simulink model "untitled"  (R2023b)
settings: Solver=VariableStepAuto  StartTime=0.0  StopTime=30  RelTol=1e-3
InitFcn:
  | clc;
  | 
  | I_xx = 228.211;
  | I_yy = 228.211;
  | I_zz = 246.355;
  | 
  | 
  | 
  | m = 327.316; %mass
  | g = 9.81; %gravitational acceleration
  | p = 1.225; %density of the environment
  | 
  | 
  | %aerodynamic forces are negligible
  | C_L = 0;
  | C_D = 0;
  | 
  | 
  | %Vector from center of gravity to the
  | %center of pressure
  | r_CP = [ 0.2; 0.0; 0.0];
  | 
  | k_r = 0.0001; %Aerodynamic damping coefficient
  | 
  | c = 20; %coefficient to calculate counter-moment
  | 
  | l = 2; %Rotor moment arm length
  | 
  | T_max = 1500; %Max thrust
  | 
  | tau = 0.05;
  | 
  | v_B = [0; 0; 0];
  | 
  | w_B = [0; 0; 0];
  | 
  | x_I = [0;0; -5];
  | 
  | euler_angles = [0;0;0];
settings Model: Creator=nijatabbasov  LastModifiedBy=nijatabbasov

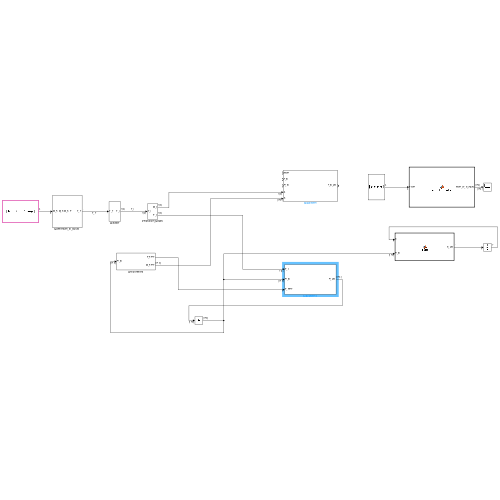
[thumbnail: Simulink's stored preview of the top-level diagram]
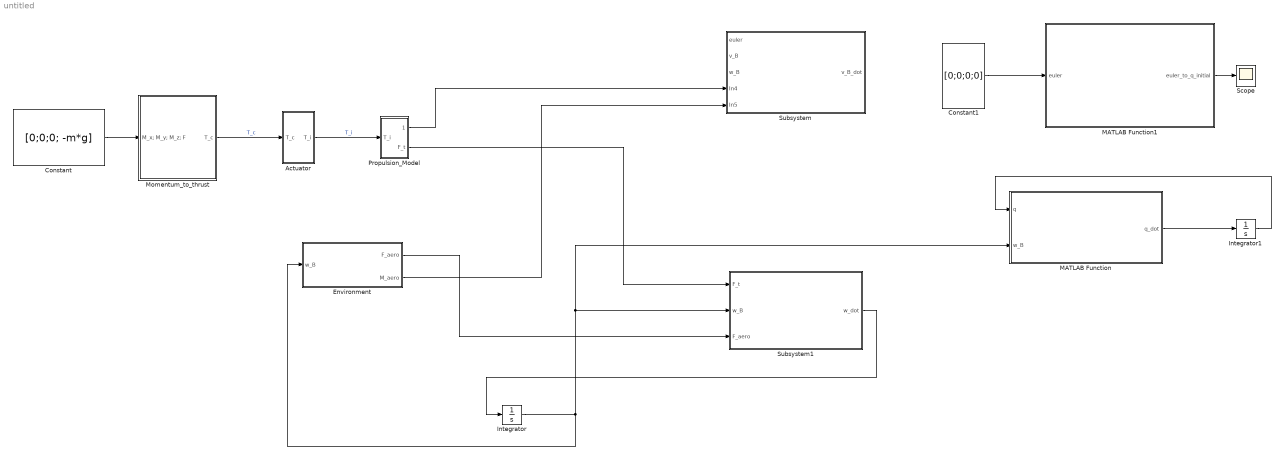
== system untitled ==
  Actuator : Subsystem
  Constant : Constant  Value=[0;0;0; -m*g]
  Constant1 : Constant  Value=[0;0;0;0]
  Environment : Subsystem
  Integrator : Integrator
  Integrator1 : Integrator
  MATLAB Function : MATLAB Function  TreatAsAtomicUnit=on
  MATLAB Function1 : MATLAB Function  TreatAsAtomicUnit=on
  "Momentum_to_thrust " : Subsystem
  Propulsion_Model : Subsystem
  Scope : Scope
  Subsystem : Subsystem
  Subsystem1 : Subsystem
  wires:
  Constant/1 -> "Momentum_to_thrust "/1(M_x; M_y; M_z; F)
  "Momentum_to_thrust "/1(T_c) -> Actuator/1(T_c)  "T_c"
  Actuator/1(T_i) -> Propulsion_Model/1(T_i)  "T_i"
  Propulsion_Model/1(M_t) -> Subsystem/4(In4)
  Environment/2(M_aero) -> Subsystem/5(In5)
  Propulsion_Model/2(F_t) -> Subsystem1/1(F_t)
  Environment/1(F_aero) -> Subsystem1/3(F_aero)
  Subsystem1/1(w_dot) -> Integrator/1
  Integrator/1 -> MATLAB Function/2(w_B), Subsystem1/2(w_B), Environment/1(w_B)
  MATLAB Function/1(q_dot) -> Integrator1/1
  Integrator1/1 -> MATLAB Function/1(q)
  Constant1/1 -> MATLAB Function1/1(euler)
  MATLAB Function1/1(euler_to_q_initial) -> Scope/1

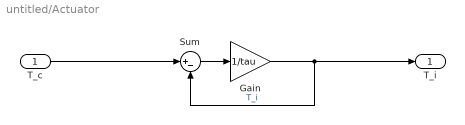
== system untitled/Actuator ==
  T_c : Inport
  Gain : Gain  Gain=1/tau
  Sum : Sum  Inputs=|+-
  T_i : Outport
  wires:
  T_c/1 -> Sum/1
  Gain/1 -> T_i/1, Sum/2  "T_i"
  Sum/1 -> Gain/1

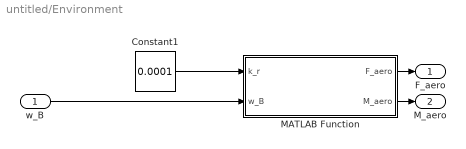
== system untitled/Environment ==
  w_B : Inport
  Constant1 : Constant  Value=0.0001
  MATLAB Function : MATLAB Function  TreatAsAtomicUnit=on
  F_aero : Outport
  M_aero : Outport  Port=2
  wires:
  w_B/1 -> MATLAB Function/2(w_B)
  MATLAB Function/2(M_aero) -> M_aero/1
  MATLAB Function/1(F_aero) -> F_aero/1
  Constant1/1 -> MATLAB Function/1(k_r)

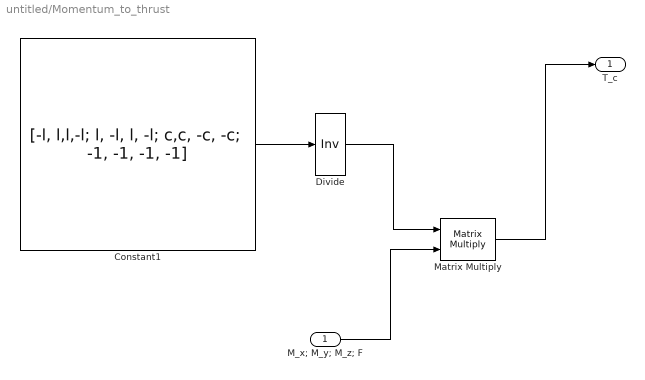
== system untitled/Momentum_to_thrust  ==
  M_x; M_y; M_z; F : Inport
  Constant1 : Constant  Value=[-l, l,l,-l; l, -l, l, -l; c,c, -c, -c; -1, -1, -1, -1]
  Divide : Product  Inputs=/  Multiplication=Matrix(*)  OutDataTypeStr=double
  Matrix Multiply : Product  Multiplication=Matrix(*)
  T_c : Outport
  wires:
  M_x; M_y; M_z; F/1 -> Matrix Multiply/2
  Matrix Multiply/1 -> T_c/1
  Divide/1 -> Matrix Multiply/1
  Constant1/1 -> Divide/1

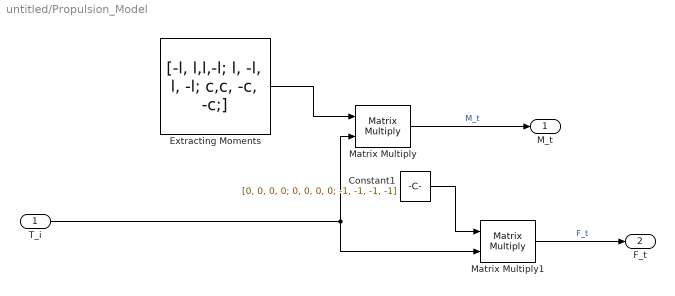
== system untitled/Propulsion_Model ==
  T_i : Inport
  Constant1 : Constant  Value=[0, 0, 0, 0; 0, 0, 0, 0; -1, -1, -1, -1]
  Extracting Moments : Constant  Value=[-l, l,l,-l; l, -l, l, -l; c,c, -c, -c;]
  Matrix Multiply : Product  Multiplication=Matrix(*)
  Matrix Multiply1 : Product  Multiplication=Matrix(*)
  M_t : Outport
  F_t : Outport  Port=2
  wires:
  T_i/1 -> Matrix Multiply1/2, Matrix Multiply/2
  Matrix Multiply/1 -> M_t/1  "M_t"
  Extracting Moments/1 -> Matrix Multiply/1
  Matrix Multiply1/1 -> F_t/1  "F_t"
  Constant1/1 -> Matrix Multiply1/1

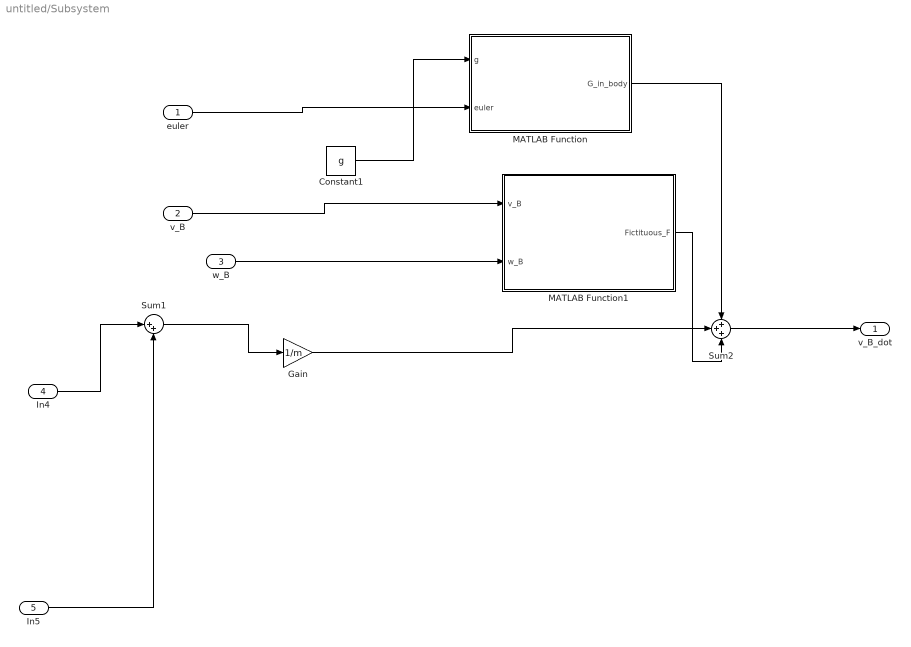
== system untitled/Subsystem ==
  euler : Inport
  v_B : Inport  Port=2
  w_B : Inport  Port=3
  In4 : Inport  Port=4
  In5 : Inport  Port=5
  Constant1 : Constant  Value=g
  Gain : Gain  Gain=1/m
  MATLAB Function : MATLAB Function  TreatAsAtomicUnit=on
  MATLAB Function1 : MATLAB Function  TreatAsAtomicUnit=on
  Sum1 : Sum  Inputs=|++
  Sum2 : Sum  Inputs=+++
  v_B_dot : Outport
  wires:
  In4/1 -> Sum1/1
  In5/1 -> Sum1/2
  w_B/1 -> MATLAB Function1/2(w_B)
  MATLAB Function/1(G_in_body) -> Sum2/1
  Constant1/1 -> MATLAB Function/1(g)
  euler/1 -> MATLAB Function/2(euler)
  MATLAB Function1/1(Fictituous_F) -> Sum2/3
  Gain/1 -> Sum2/2
  v_B/1 -> MATLAB Function1/1(v_B)
  Sum2/1 -> v_B_dot/1
  Sum1/1 -> Gain/1

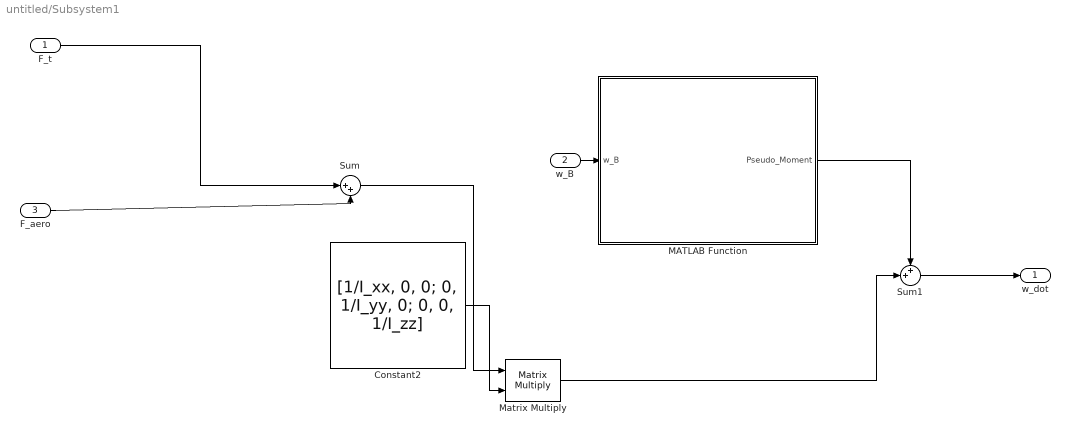
== system untitled/Subsystem1 ==
  F_t : Inport
  w_B : Inport  Port=2
  F_aero : Inport  Port=3
  Constant2 : Constant  Value=[1/I_xx, 0, 0; 0, 1/I_yy, 0; 0, 0, 1/I_zz]
  MATLAB Function : MATLAB Function  TreatAsAtomicUnit=on
  Matrix Multiply : Product  Multiplication=Matrix(*)
  Sum : Sum  Inputs=|++
  Sum1 : Sum  Inputs=++|
  w_dot : Outport
  wires:
  F_t/1 -> Sum/1
  Matrix Multiply/1 -> Sum1/2
  w_B/1 -> MATLAB Function/1(w_B)
  Constant2/1 -> Matrix Multiply/2
  Sum1/1 -> w_dot/1
  F_aero/1 -> Sum/2
  Sum/1 -> Matrix Multiply/1
  MATLAB Function/1(Pseudo_Moment) -> Sum1/1

== matlab function untitled/Subsystem/MATLAB Function ==
  data: g input; G_in_body output; euler input
function G_in_body = G_in_body(g, euler)
    % This function evaluates derivative of vehicle speed in body frame 
    % and angular velocity of the center of gravity of the vehicle
    %Acceler is (F_thrust + F_aero)/m
    phi = euler(1);
    theta = euler(2);
    

    
    frame_change = [-sin(theta); sin(phi)*cos(theta); cos(phi)* cos(theta)];


    G_in_body = frame_change * g;
   
end

== matlab function untitled/Environment/MATLAB Function ==
  data: k_r input; F_aero output; w_B input; M_aero output
function [F_aero, M_aero] = F_aero_M_aero(k_r, w_B)

    F_aero = 0;
    M_aero = - k_r * w_B;

== matlab function untitled/Subsystem/MATLAB Function1 ==
  data: v_B input; Fictituous_F output; w_B input
function Fictituous_F = Fictituous_F(v_B, w_B)
    % This function evaluates derivative of vehicle speed in body frame 
    % and angular velocity of the center of gravity of the vehicle
    
    p = w_B(1);
    q = w_B(2);
    r = w_B(3);


    w_x = [0, -r,  q;
           r,  0, -p;
          -1   p   0   ];

   

    Fictituous_F = w_x * v_B;
    
end

== matlab function untitled/Subsystem1/MATLAB Function ==
  data: w_B input; Pseudo_Moment output
function Pseudo_Moment = Pseudo_Moment(w_B)
    % This function evaluates value of w*(Iw)
   
    p = w_B(1);
    q = w_B(2);
    r = w_B(3);


    
    
   
    I_xx = 228.211; 
    I_yy = 228.211;
    I_zz = 246.355;



    Pseudo_Moment = [(I_yy-I_zz)*q*r/I_xx; (I_zz - I_xx)*p*r/I_yy; (I_xx - I_yy)*p*q/I_zz];
   
    
end

== matlab function untitled/MATLAB Function ==
  data: q input; q_dot output; w_B input
function q_dot = q_dot(q, w_B)
    q_0 = q(1);
    q_1 = q(2);
    q_2 = q(3);
    q_3 = q(4);

    p = w_B(1);
    q = w_B(2);
    r = w_B(3);

    epsilon_q = 1-(q_0^2 + q_1^2 + q_2^2 + q_3^2);

    C_k = 5;
    A = [0, -p, -q, -r;
         p,  0,  r, -q;
         q, -r,  0,  p;
         r,  q, -p,  0];

    
    q_dot = 1/2 * A *q + C_k * epsilon_q*q;


end

== matlab function untitled/MATLAB Function1 ==
  data: euler input; euler_to_q_initial output
function euler_to_q_initial = euler_to_q_initial(euler)

    phi = euler(1); 
    theta = euler(2); 
    psi = euler(3);


    phi = deg2rad(phi);
    theta = deg2rad(theta);
    psi = deg2rad(psi);

    q0 = cos(psi/2)*cos(theta/2)*cos(phi/2) + sin(psi/2)*sin(theta/2)*sin(phi/2);
    q1 = cos(psi/2)*cos(theta/2)*sin(phi/2) - sin(psi/2)*sin(theta/2)*cos(phi/2);
    q2 = cos(psi/2)*sin(theta/2)*cos(phi/2) + sin(psi/2)*cos(theta/2)*sin(phi/2);
    q3 = sin(psi/2)*cos(theta/2)*cos(phi/2) - cos(psi/2)*sin(theta/2)*sin(phi/2);


    euler_to_q_initial= [q0, q1, q2, q3];

end
